simulink model "P_2_1_f_Egyszeru_kocsi_modell"  (R2021b)
settings: Solver=ode4  StartTime=0.0  StopTime=50  FixedStep=0.01  RelTol=1e-3
settings Model: Creator=davidpaksi  LastModifiedBy=davidpaksi

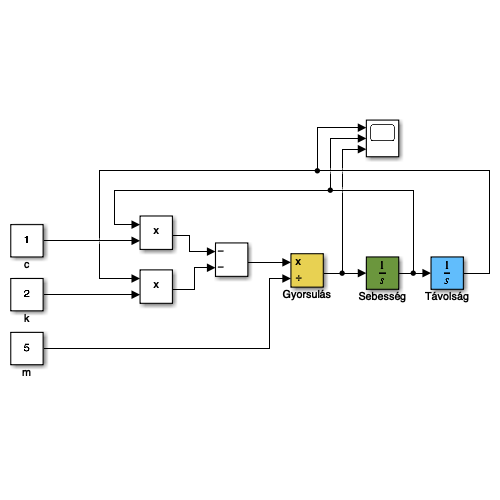
[thumbnail: Simulink's stored preview of the top-level diagram]
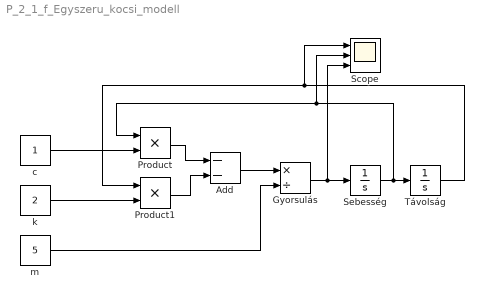
== system P_2_1_f_Egyszeru_kocsi_modell ==
  Add : Sum  Inputs=--
  Gyorsulás : Product  Inputs=*/
  Product : Product
  Product1 : Product
  Scope : Scope  NumInputPorts=3
  Sebesség : Integrator
  Távolság : Integrator  InitialCondition=1
  c : Constant
  k : Constant  Value=2
  m : Constant  Value=5
  wires:
  Sebesség/1 -> Product/1, Scope/2, Távolság/1
  Gyorsulás/1 -> Scope/3, Sebesség/1
  Add/1 -> Gyorsulás/1
  Product/1 -> Add/1
  Product1/1 -> Add/2
  Távolság/1 -> Product1/1, Scope/1
  c/1 -> Product/2
  k/1 -> Product1/2
  m/1 -> Gyorsulás/2
